simulink model "FullConrle"  (Simulink 7.5)
settings: Solver=ode23tb  StartTime=0.0  StopTime=10  RelTol=1e-3
libraries: powerlib x12
settings Model: Creator=ninad gaikawad  LastModifiedBy=ninad gaikawad

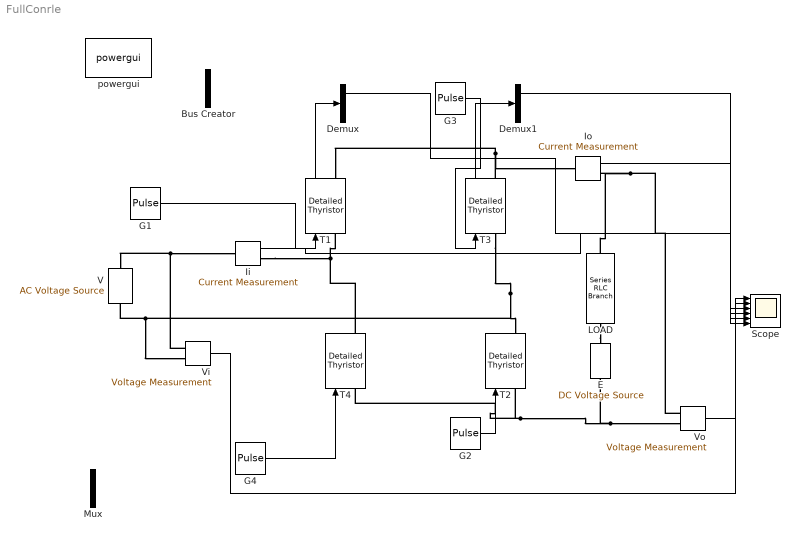
== system FullConrle ==
  " T1" : powerlib/Power Electronics/Detailed Thyristor  DialogController=POWERSYS.PowerSysDialog  SystemSampleTime=-1  Ron=0.001  Lon=1e-3  Vf=0.8  IL=0.1  Tq=100e-6  IC=0  Rs=500  Cs=250e-9  Measurements=on
  Bus Creator : BusCreator  Inputs=2
  Demux : Demux  Outputs=2
  Demux1 : Demux  Outputs=2
  E : powerlib/Electrical Sources/DC Voltage Source  DialogController=POWERSYS.PowerSysDialog  SystemSampleTime=-1  Amplitude=100  Measurements=None
  G1 : DiscretePulseGenerator  PulseType=Time based  Amplitude=1  Period=20*10^(-3)  PulseWidth=5  PhaseDelay=3*10^(-3)  SampleTime=1
  G2 : DiscretePulseGenerator  PulseType=Time based  Amplitude=1  Period=20*10^(-3)  PulseWidth=5  PhaseDelay=3*10^(-3)  SampleTime=1
  G3 : DiscretePulseGenerator  PulseType=Time based  Amplitude=1  Period=20*10^(-3)  PulseWidth=5  PhaseDelay=13*10^(-3)  SampleTime=1
  G4 : DiscretePulseGenerator  PulseType=Time based  Amplitude=1  Period=20*10^(-3)  PulseWidth=5  PhaseDelay=13*10^(-3)  SampleTime=1
  Ii : powerlib/Measurements/Current Measurement  DialogController=POWERSYS.PowerSysDialog  SystemSampleTime=-1  PhasorSimulation=off  OutputType=Complex  PSBequivalent=0
  Io : powerlib/Measurements/Current Measurement  DialogController=POWERSYS.PowerSysDialog  SystemSampleTime=-1  PhasorSimulation=off  OutputType=Complex  PSBequivalent=0
  LOAD : powerlib/Elements/Series RLC Branch  DialogController=POWERSYS.PowerSysDialog  PhysicalDomain=powersysdomain  SubClassName=unknown  LeftPortType=p1  RightPortType=p1  LConnTagsString=__new0  RConnTagsString=__new0  BranchType=RL  Resistance=10  Inductance=1  SetiL0=off  InitialCurrent=0  Capacitance=1e-6  Setx0=off  InitialVoltage=0  Measurements=None
  Mux : Mux  Inputs=2
  Scope : Scope  NumInputPorts=6
      settings: YMin=-5~-5~-5~-5~-5~-5  YMax=5~5~5~5~5~5
  T2 : powerlib/Power Electronics/Detailed Thyristor  DialogController=POWERSYS.PowerSysDialog  SystemSampleTime=-1  Ron=0.001  Lon=1e-3  Vf=0.8  IL=0.1  Tq=100e-6  IC=0  Rs=500  Cs=250e-9  Measurements=on
  T3 : powerlib/Power Electronics/Detailed Thyristor  DialogController=POWERSYS.PowerSysDialog  SystemSampleTime=-1  Ron=0.001  Lon=1e-3  Vf=0.8  IL=0.1  Tq=100e-6  IC=0  Rs=500  Cs=250e-9  Measurements=on
  T4 : powerlib/Power Electronics/Detailed Thyristor  DialogController=POWERSYS.PowerSysDialog  SystemSampleTime=-1  Ron=0.001  Lon=1e-3  Vf=0.8  IL=0.1  Tq=100e-6  IC=0  Rs=500  Cs=250e-9  Measurements=on
  V : powerlib/Electrical Sources/AC Voltage Source  DialogController=POWERSYS.PowerSysDialog  SystemSampleTime=-1  Amplitude=325.23  Phase=0  Frequency=50  SampleTime=0  Measurements=None
  Vi : powerlib/Measurements/Voltage Measurement  DialogController=POWERSYS.PowerSysDialog  SystemSampleTime=-1  PhasorSimulation=off  OutputType=Complex  PSBequivalent=0
  Vo : powerlib/Measurements/Voltage Measurement  DialogController=POWERSYS.PowerSysDialog  SystemSampleTime=-1  PhasorSimulation=off  OutputType=Complex  PSBequivalent=0
  powergui : powerlib/powergui  Priority=1  SystemSampleTime=-1  SimulationMode=Continuous  SampleTime=50e-6  frequency=60  SPID=off  DisableSnubberDevices=off  DisableRonSwitches=off  DisableVfSwitches=off  SwTol=0  Interpol=off  frequencyindice=50  echomessages=off  HookPort=off  DisplayEquations=off  FunctionMessages=off  EnableUseOfTLC=off  x0status=blocks  RestoreLinks=warning  ResistiveCurrentMeasurement=off  Ylog=off  Xlog=on  ShowGrid=off  save=off  variable=ZData  ZoomFFT=off  StartTime=0.0  cycles=1  DisplayStyle=1  FreqAxis=off  MaxFrequency=1000  frequencyindicesteady=1  display=off  methode=off
  wires:
  G4/1 -> T4/1
  G1/1 -> " T1"/1
  G2/1 -> T2/1
  G3/1 -> T3/1
  T3/1 -> Demux1/1
  " T1"/1 -> Demux/1
  Vi/1 -> Scope/1
  Vo/1 -> Scope/2
  Io/1 -> Scope/3
  Ii/1 -> Scope/4
  Demux/1 -> Scope/5
  Demux1/1 -> Scope/6
  connections:
  Vi/LConn1 -- V/RConn1 -- Ii/LConn1
  T2/LConn1 -- T4/LConn1 -- Vo/LConn2 -- E/LConn1
  T2/RConn1 -- V/LConn1 -- Vi/LConn2 -- T3/LConn1
  T3/RConn1 -- Io/LConn1 -- " T1"/RConn1
  Vo/LConn1 -- Io/RConn1 -- LOAD/RConn1
  T4/RConn1 -- " T1"/LConn1 -- Ii/RConn1
  LOAD/LConn1 -- E/RConn1
